simulink model "Practica7simulink"  (R2024b)
settings: Solver=VariableStepAuto  StartTime=0.0  StopTime=2  RelTol=1e-3
InitFcn:
  | R=5000000;
  | C=100*10^-9;
  | U=5;
undefined symbols (not defined in the file or in its folder): c1, c2, r1, r2, r3
settings Model: Creator=sanch

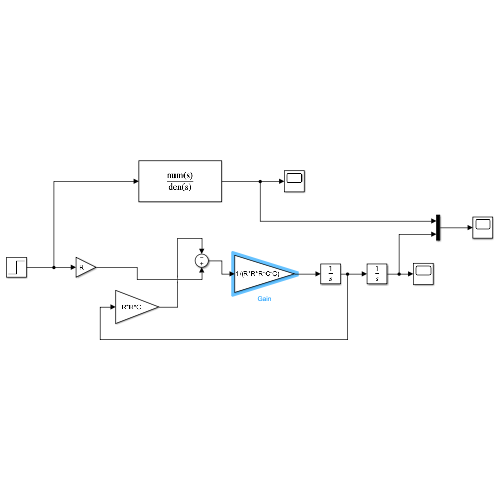
[thumbnail: Simulink's stored preview of the top-level diagram]
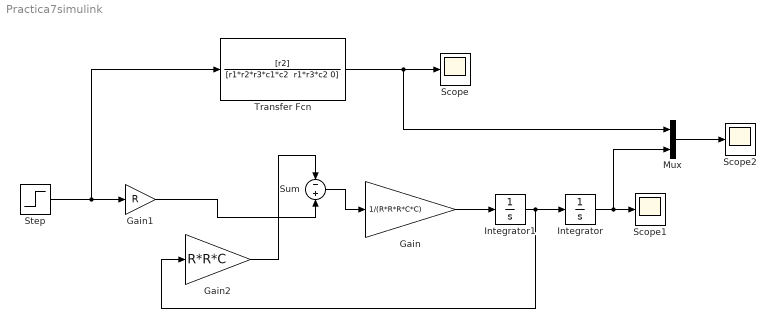
== system Practica7simulink ==
  Gain : Gain  Gain=1/(R*R*R*C*C)
  Gain1 : Gain  Gain=R
  Gain2 : Gain  Gain=R*R*C
  Integrator : Integrator
  Integrator1 : Integrator
  Mux : Mux  Inputs=2
  Scope : Scope
  Scope1 : Scope
  Scope2 : Scope
  Step : Step  SampleTime=0
  Sum : Sum  Inputs=-+
  Transfer Fcn : TransferFcn  Numerator=[r2]  Denominator="[r1*r2*r3*c1*c2  r1*r3*c2 0]"
  wires:
  Step/1 -> Transfer Fcn/1, Gain1/1
  Gain2/1 -> Sum/1
  Gain1/1 -> Sum/2
  Transfer Fcn/1 -> Mux/1, Scope/1
  Sum/1 -> Gain/1
  Mux/1 -> Scope2/1
  Gain/1 -> Integrator1/1
  Integrator/1 -> Mux/2, Scope1/1
  Integrator1/1 -> Gain2/1, Integrator/1
